simulink model "comm_test"  (R2022a)
settings: Solver=FixedStepAuto  StartTime=0.0  StopTime=10.0  RelTol=1e-3  EnableMultiTasking=on
libraries: hdlsllib x4, simulink x3, mbedblockslib x2
settings Model: ExtModeTrigDuration=10  Creator=FUGAZI  LastModifiedBy=smith
settings OptimizationCC: EnhancedBackFolding=on  PassReuseOutputArgsAs=Individual arguments  ZeroExternalMemoryAtStartup=off  ZeroInternalMemoryAtStartup=off  MaxStackSize=64  OptimizeBlockOrder=speed  DifferentSizesBufferReuse=on  OptimizationCustomize=off  EfficientTunableParamExpr=on
settings DebuggingCC: ParameterTunabilityLossMsg=error
settings HardwareCC: ProdBitPerPointer=32  ProdBitPerSizeT=32  ProdBitPerPtrDiffT=32  ProdLargestAtomicInteger=Long  ProdLargestAtomicFloat=Double  ProdWordSize=32  ProdLongLongMode=on  ProdHWDeviceType=ARM Compatible->ARM Cortex
settings SFSimCC: MATLABDynamicMemAlloc=off
settings RTWCC: SystemTargetFile=ert.tlc  HardwareBoard=STM32 Nucleo L476RG  TemplateMakefile=ert_default_tmf  Toolchain=GNU Tools for ARM Embedded Processors
settings CodeAppCC: ForceParamTrailComments=on  IgnoreCustomStorageClasses=off  OperatorAnnotations=on  SimulinkDataObjDesc=on  SFDataObjDesc=on  InsertBlockDesc=on
settings ERTTargetCC: ExtModeTransport=3  ExtModeStaticAlloc=on  ExtModeStaticAllocSize=2000  ExtModeMexFile=ext_xcp  ExtModeIntrfLevel=Level2 - Open

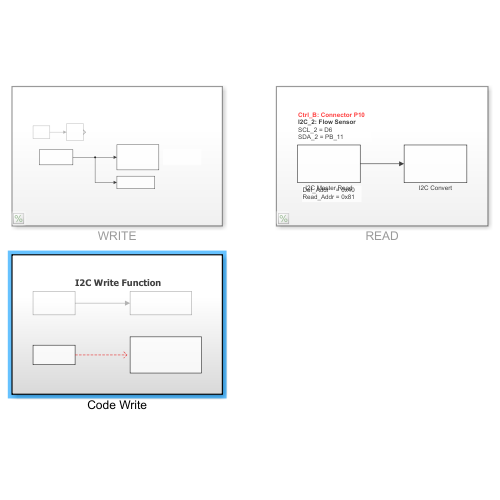
[thumbnail: Simulink's stored preview of the top-level diagram]
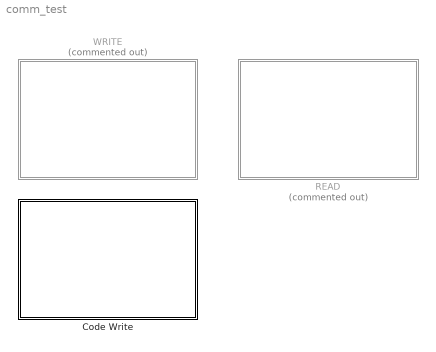
== system comm_test ==
  Code Write : Subsystem
  READ : Subsystem  Commented=on
  WRITE : Subsystem  Commented=on

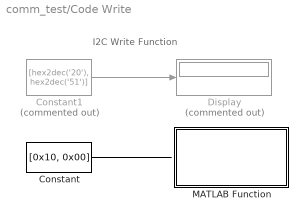
== system comm_test/Code Write ==
  note: I2C Write Function
  Constant : Constant  Value=[0x10, 0x00]
  Constant1 : Constant  Commented=on  Value=[hex2dec('20'), hex2dec('51')]
  Display : Display  Commented=on
  MATLAB Function : MATLAB Function  TreatAsAtomicUnit=on
  wires:
  Constant/1 -> ?
  Constant1/1 -> Display/1

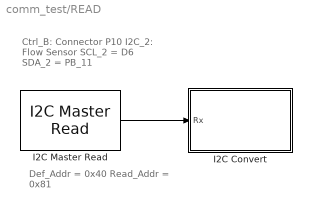
== system comm_test/READ ==
  note: Def_Addr = 0x40
      | Read_Addr = 0x81
  note: Ctrl_B: Connector P10
      | I2C_2: Flow Sensor
      | SCL_2 = D6
      | SDA_2 = PB_11
  I2C Convert : Subsystem
  I2C Master Read : mbedblockslib/I2C Master Read  I2CModule=0  Mode=Master  SlaveAddress=hex2dec('80')  SlaveByteOrder=BigEndian  Direction=Receiver  RegisterAddressMode=off  RegisterAddress=uint8(0)  SlaveDataType=uint8  DataLength=3  NoAck=on  RepeatedStart=on  OutputStatus=off  SampleTime=0.1
      settings: SourceProductBaseCode=MICROBIT,NUCLEO,STMICRODIS
  wires:
  I2C Master Read/1 -> I2C Convert/1(Rx)

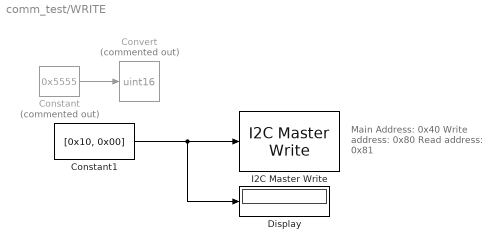
== system comm_test/WRITE ==
  note: Main Address: 0x40
      | Write address: 0x80
      | Read address: 0x81
  Constant : Constant  Commented=on  Value=0x5555  SampleTime=0.1
  Constant1 : Constant  Value=[0x10, 0x00]
  Convert : DataTypeConversion  Commented=on  OutDataTypeStr=uint16  RndMeth=Nearest  SaturateOnIntegerOverflow=off
  Display : Display
      settings: Format=hex (Stored Integer)
  I2C Master Write : mbedblockslib/I2C Master Write  I2CModule=0  Mode=Master  SlaveAddress=hex2dec('40')  SlaveByteOrder=BigEndian  Direction=Transmitter  RegisterAddressMode=off  RegisterAddress=uint8(1)  SlaveDataType=uint8  DataLength=2  NoAck=off  RepeatedStart=on  OutputStatus=off
      settings: SourceProductBaseCode=MICROBIT,NUCLEO,STMICRODIS
  wires:
  Constant/1 -> Convert/1
  Constant1/1 -> Display/1, I2C Master Write/1

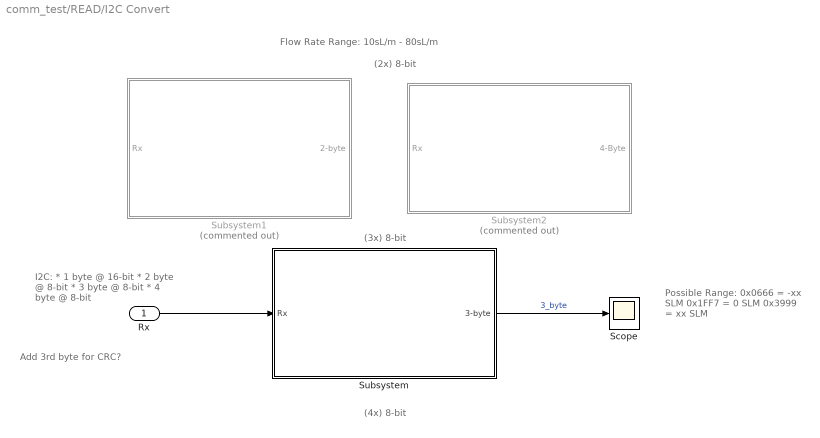
== system comm_test/READ/I2C Convert ==
  note: (2x) 8-bit
  note: Possible Range:
      | 0x0666 = -xx SLM
      | 0x1FF7 = 0 SLM
      | 0x3999 = xx SLM
  note: Flow Rate Range: 10sL/m - 80sL/m
  note: I2C:
      | * 1 byte @ 16-bit
      | * 2 byte @ 8-bit
      | * 3 byte @ 8-bit
      | * 4 byte @ 8-bit
  note: Add 3rd byte for CRC?
  note: (3x) 8-bit
  note: (4x) 8-bit
  Rx : Inport
  Scope : Scope
  Subsystem : Subsystem
  Subsystem1 : Subsystem  Commented=on
  Subsystem2 : Subsystem  Commented=on
  wires:
  Rx/1 -> Subsystem/1(Rx)
  Subsystem/1(3-byte) -> Scope/1  "3_byte"

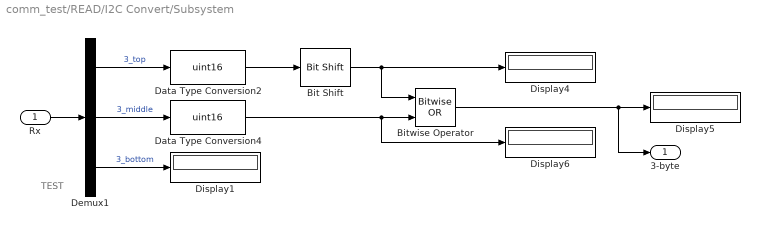
== system comm_test/READ/I2C Convert/Subsystem ==
  note: TEST
  Rx : Inport
  Bit Shift : hdlsllib/Logic and Bit Operations/Bit Shift  mode=Shift Left Logical  N=8
  Bitwise Operator : simulink/Logic and Bit Operations/Bitwise Operator  logicop=OR  UseBitMask=off  NumInputPorts=2  BitMask=bin2dec('11011001')  BitMaskRealWorld=Stored Integer
  Data Type Conversion2 : DataTypeConversion  OutDataTypeStr=uint16  SaturateOnIntegerOverflow=off  RndMeth=Floor
  Data Type Conversion4 : DataTypeConversion  OutDataTypeStr=uint16  SaturateOnIntegerOverflow=off  RndMeth=Floor
  Demux1 : Demux  Outputs=3
  Display{1,4..6} (4 alike) : Display
      settings: Format=hex (Stored Integer)
  3-byte : Outport
  wires:
  Bit Shift/1 -> Bitwise Operator/1, Display4/1
  Data Type Conversion4/1 -> Display6/1, Bitwise Operator/2
  Bitwise Operator/1 -> 3-byte/1, Display5/1
  Data Type Conversion2/1 -> Bit Shift/1
  Rx/1 -> Demux1/1
  Demux1/1 -> Data Type Conversion2/1  "3_top"
  Demux1/2 -> Data Type Conversion4/1  "3_middle"
  Demux1/3 -> Display1/1  "3_bottom"

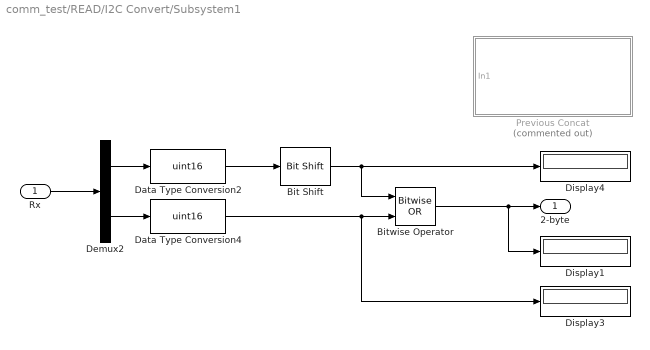
== system comm_test/READ/I2C Convert/Subsystem1 ==
  Rx : Inport
  Bit Shift : hdlsllib/Logic and Bit Operations/Bit Shift  mode=Shift Left Logical  N=8
  Bitwise Operator : simulink/Logic and Bit Operations/Bitwise Operator  logicop=OR  UseBitMask=off  NumInputPorts=2  BitMask=bin2dec('11011001')  BitMaskRealWorld=Stored Integer
  Data Type Conversion2 : DataTypeConversion  OutDataTypeStr=uint16  SaturateOnIntegerOverflow=off  RndMeth=Floor
  Data Type Conversion4 : DataTypeConversion  OutDataTypeStr=uint16  SaturateOnIntegerOverflow=off  RndMeth=Floor
  Demux2 : Demux  Outputs=2
  Display1 : Display
      settings: Format=hex (Stored Integer)
  Display3 : Display
      settings: Format=hex (Stored Integer)
  Display4 : Display
      settings: Format=hex (Stored Integer)
  Previous Concat : Subsystem  Commented=on
  2-byte : Outport
  wires:
  Rx/1 -> Demux2/1
  Demux2/1 -> Data Type Conversion2/1
  Data Type Conversion2/1 -> Bit Shift/1
  Bit Shift/1 -> Display4/1, Bitwise Operator/1
  Data Type Conversion4/1 -> Display3/1, Bitwise Operator/2
  Demux2/2 -> Data Type Conversion4/1
  Bitwise Operator/1 -> Display1/1, 2-byte/1

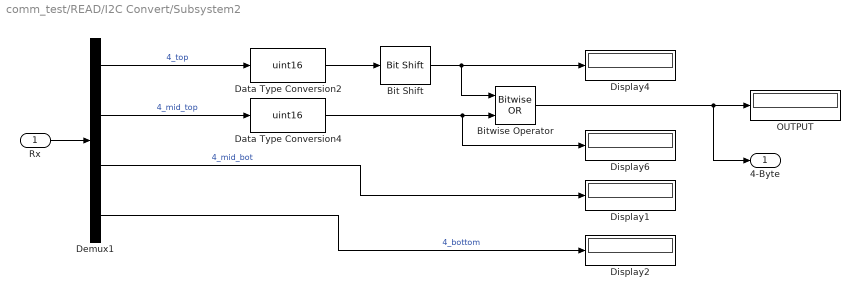
== system comm_test/READ/I2C Convert/Subsystem2 ==
  Rx : Inport
  Bit Shift : hdlsllib/Logic and Bit Operations/Bit Shift  mode=Shift Left Logical  N=8
  Bitwise Operator : simulink/Logic and Bit Operations/Bitwise Operator  logicop=OR  UseBitMask=off  NumInputPorts=2  BitMask=bin2dec('11011001')  BitMaskRealWorld=Stored Integer
  Data Type Conversion2 : DataTypeConversion  OutDataTypeStr=uint16  SaturateOnIntegerOverflow=off  RndMeth=Floor
  Data Type Conversion4 : DataTypeConversion  OutDataTypeStr=uint16  SaturateOnIntegerOverflow=off  RndMeth=Floor
  Demux1 : Demux
  Display{1..2,4,6} (4 alike) : Display
      settings: Format=hex (Stored Integer)
  OUTPUT : Display
      settings: Format=hex (Stored Integer)
  4-Byte : Outport
  wires:
  Data Type Conversion2/1 -> Bit Shift/1
  Bitwise Operator/1 -> 4-Byte/1, OUTPUT/1
  Bit Shift/1 -> Display4/1, Bitwise Operator/1
  Demux1/4 -> Display2/1  "4_bottom"
  Rx/1 -> Demux1/1
  Demux1/2 -> Data Type Conversion4/1  "4_mid_top"
  Demux1/1 -> Data Type Conversion2/1  "4_top"
  Data Type Conversion4/1 -> Display6/1, Bitwise Operator/2
  Demux1/3 -> Display1/1  "4_mid_bot"

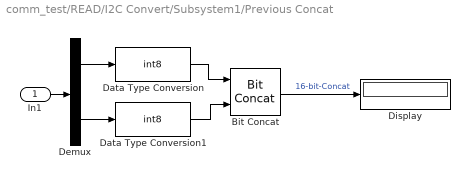
== system comm_test/READ/I2C Convert/Subsystem1/Previous Concat ==
  In1 : Inport
  Bit Concat : hdlsllib/Logic and Bit Operations/Bit Concat  numInputs=2
  Data Type Conversion : DataTypeConversion  OutDataTypeStr=int8  SaturateOnIntegerOverflow=off  RndMeth=Floor
  Data Type Conversion1 : DataTypeConversion  OutDataTypeStr=int8  SaturateOnIntegerOverflow=off  RndMeth=Floor
  Demux : Demux  Outputs=2
  Display : Display
      settings: Format=hex (Stored Integer)
  wires:
  Data Type Conversion/1 -> Bit Concat/1
  Bit Concat/1 -> Display/1  "16-bit-Concat"
  Demux/2 -> Data Type Conversion1/1
  Data Type Conversion1/1 -> Bit Concat/2
  Demux/1 -> Data Type Conversion/1
  In1/1 -> Demux/1

== matlab function comm_test/Code Write/MATLAB Function ==

function writeByteToSTM32()
    %arduinoObj = arduino('COM3','Uno','Libraries','I2C');  % ERROR

    board =  'NUCLEO-L476RG';                               % Options: nucleo; / nucleo('COM4');
    %pinMode = configurePin(board,'P10');                   % Get pin config - ERROR
    configurePin(board, 'D14', 'I2C SDA');                  % ERROR: undefined
    configurePin(board, 'D15', 'I2C SCL');                  % ERROR: undefined

    deviceAddress = hex2dec('40');
    byteToWrite = hex2dec('10');

    writeRegister(board, deviceAddress, byteToWrite);       % ERROR: undefined
end
